simulink model "ramp"  (Simulink 7.5)
settings: Solver=ode45  StartTime=0.0  StopTime=inf  RelTol=1e-3
undefined symbols (not defined in the file or in its folder): Columns
libraries: dspsigops x1, simulink x1
settings Model: Creator=Mircea  LastModifiedBy=Mircea

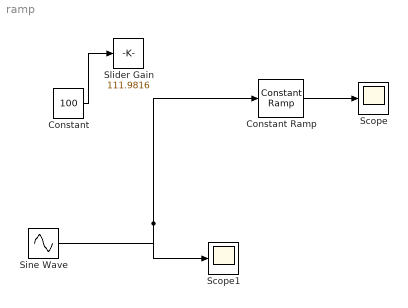
== system ramp ==
  Constant : Constant  Value=100  OutDataType=fixdt(1, 16)  OutScaling=2^0
  Constant Ramp : dspsigops/Constant Ramp  L=Columns  dim=1  Slope=2  dataType=single  isSigned=on  wordLen=16  udDataType=sfix(16)  fracBitsMode=Best precision  numFracBits=15  Offset=0
  Scope : Scope
      settings: YMin=-1  YMax=1
  Scope1 : Scope
      settings: YMin=-72.22  YMax=-72.135
  Sine Wave : Sin  Amplitude=111  Bias=0  Frequency=0.0001  Phase=0  Samples=10  SampleTime=0  Offset=0
  Slider Gain : simulink/Math Operations/Slider Gain  SystemSampleTime=-1  low=-180  gain=111.9816  high=180
  wires:
  Constant/1 -> Slider Gain/1
  Constant Ramp/1 -> Scope/1
  Sine Wave/1 -> Constant Ramp/1, Scope1/1
